simulink model "FMC_StateMachineNew"  (R2025a)
settings: Solver=VariableStepAuto  StartTime=0.0  StopTime=10.0  RelTol=1e-3
libraries: simulink x1
settings Model: Creator=ro23498  LastModifiedBy=ro23498

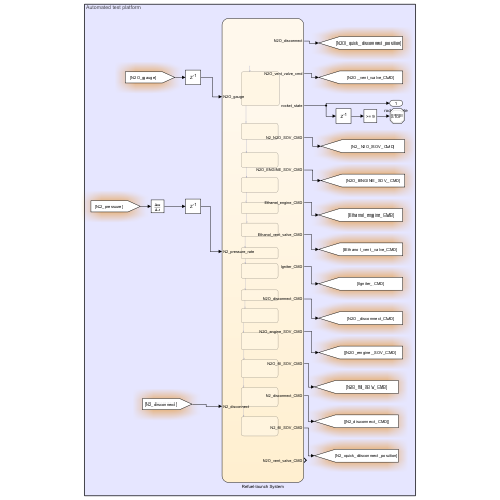
[thumbnail: Simulink's stored preview of the top-level diagram]
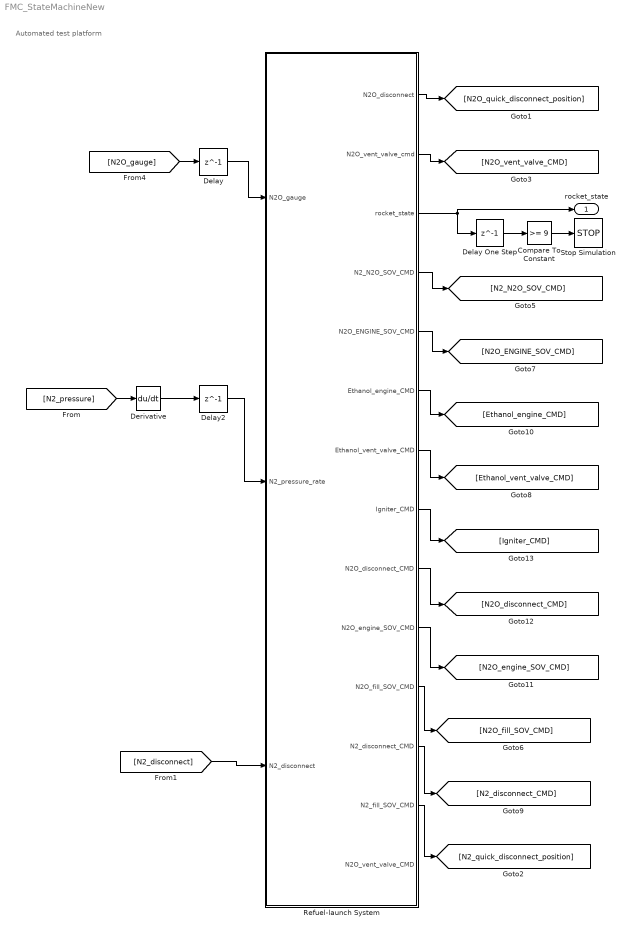
== system FMC_StateMachineNew ==
  note: Automated test platform
  Compare To Constant : simulink/Logic and Bit Operations/Compare To Constant  relop=>=  const=9  OutDataTypeStr=boolean
  Delay : Delay  DelayLength=1
  Delay One Step : Delay  DelayLength=1
  Delay2 : Delay  DelayLength=1
  Derivative : Derivative
  Refuel-launch System : Stateflow chart  TreatAsAtomicUnit=on  SystemSampleTime=0.5
  Stop Simulation : Stop
  rocket_state : Outport
  wires:
  [N2O_gauge] -> Delay/1
  Delay/1 -> Refuel-launch System/1(N2O_gauge)
  [N2_pressure] -> Derivative/1
  Derivative/1 -> Delay2/1
  Delay2/1 -> Refuel-launch System/2(N2_pressure_rate)
  Refuel-launch System/1(N2O_disconnect) -> [N2O_quick_disconnect_position]
  Refuel-launch System/2(N2O_vent_valve_cmd) -> [N2O_vent_valve_CMD]
  Refuel-launch System/3(rocket_state) -> Delay One Step/1, rocket_state/1
  Delay One Step/1 -> Compare To Constant/1
  Compare To Constant/1 -> Stop Simulation/1
  Refuel-launch System/5(N2O_ENGINE_SOV_CMD) -> [N2O_ENGINE_SOV_CMD]
  Refuel-launch System/4(N2_N2O_SOV_CMD) -> [N2_N2O_SOV_CMD]
  Refuel-launch System/6(Ethanol_engine_CMD) -> [Ethanol_engine_CMD]
  Refuel-launch System/7(Ethanol_vent_valve_CMD) -> [Ethanol_vent_valve_CMD]
  Refuel-launch System/12(N2_disconnect_CMD) -> [N2_disconnect_CMD]
  Refuel-launch System/8(Igniter_CMD) -> [Igniter_CMD]
  Refuel-launch System/9(N2O_disconnect_CMD) -> [N2O_disconnect_CMD]
  Refuel-launch System/13(N2_fill_SOV_CMD) -> [N2_quick_disconnect_position]
  Refuel-launch System/11(N2O_fill_SOV_CMD) -> [N2O_fill_SOV_CMD]
  Refuel-launch System/10(N2O_engine_SOV_CMD) -> [N2O_engine_SOV_CMD]
  [N2_disconnect] -> Refuel-launch System/3(N2_disconnect)

== stateflow chart FMC_StateMachineNew/Refuel-launch System ==
  state IDLE
    en:
    rocket_state = 0;
    N2O_disconnect_CMD = 0;
    N2_disconnect_CMD = 0;
    N2O_vent_valve_CMD = 0;
    Ethanol_vent_valve_CMD = 0;
    N2O_fill_SOV_CMD = 0;
    N2_fill_SOV_CMD = 0;
    N2O_engine_SOV_CMD = 0;
    Ethanol_engine_CMD = 0;
    Igniter_CMD = 0;
  state N2O_refueling
    en:
    rocket_state = 1;
    N2O_disconnect_CMD = 1;
    N2O_fill_SOV_CMD = 1;
  state N2O_refueling_complete
    en:
    rocket_state = 2;
    N2O_disconnect_CMD = 0;
    N2O_fill_SOV_CMD = 0;
  state N2O_pressurizing
    en:
    rocket_state = 3;
    N2_disconnect_CMD = 1;
    N2_fill_SOV_CMD = 1;
  state pressurization_check
    en:
    rocket_state=4;
  state N2_refueling
    en:
    N2_disconnect = 1;
    rocket_state = 3;
  state check_progress
    en:
  state N2_refueling_complete
    en:
    N2_disconnect = 0;
    rocket_state = 4;
  state Refuel_complete
    en:
    rocket_state = 5;
  state Ignition_precondition
    en:
    rocket_state = 5.5;
    N2_N2O_SOV_CMD = 1;
  state Launch
    en:
    rocket_state = 6;
    N2_N2O_SOV_CMD = 1;
    N2O_ENGINE_SOV_CMD = 1;
    Ethanol_engine_CMD = 1;
  state MECO
    en:
    rocket_state = 7;
    N2_N2O_SOV_CMD = 0;
    N2O_ENGINE_SOV_CMD = 0;
    Ethanol_engine_CMD = 0;
  state Start_vent
    en:
    rocket_state = 8;
    Ethanol_vent_valve_CMD = 1;
    N2O_vent_valve_cmd = 1;
  state Vent_complete
    en:
    rocket_state = 9;
    Ethanol_vent_valve_CMD = 0;
    N2O_vent_valve_cmd = 0;
  (default) -> IDLE
  IDLE -> N2O_refueling
  N2O_refueling -> N2O_refueling_complete : [N2O_gauge >= dipstick_gauge_start]
  N2O_refueling_complete -> N2O_pressurizing : after(60, sec)
  N2O_pressurizing -> pressurization_check
  pressurization_check -> N2_refueling
  N2_refueling -> check_progress : after(60, sec)
  check_progress -> N2_refueling_complete : [N2_pressure_rate<0.01]
  N2_refueling_complete -> Refuel_complete
  Refuel_complete -> Ignition_precondition : after(12000, sec)
  Ignition_precondition -> Launch : after(10, sec)
  Launch -> MECO : after(4.5, sec)
  MECO -> Start_vent : after(1, sec)
  Start_vent -> Vent_complete : after(5, sec)
  data: N2O_disconnect output; N2O_vent_valve_cmd output; dipstick_gauge_start parameter; N2O_gauge input; N2_pressure_rate input; rocket_state output; N2_N2O_SOV_CMD output; N2O_ENGINE_SOV_CMD output; Ethanol_engine_CMD output; Ethanol_vent_valve_CMD output; Igniter_CMD output; N2O_disconnect_CMD output; N2O_engine_SOV_CMD output; N2O_fill_SOV_CMD output; N2_disconnect_CMD output; N2_fill_SOV_CMD output; N2_disconnect input; N2O_vent_valve_CMD output
